simulink model "Q1_2_2"  (R2020b)
settings: Solver=VariableStepAuto  StartTime=0.0  StopTime=20.0  RelTol=1e-3
libraries: simulink x2
settings Model: Creator=kushagrakhatwani  LastModifiedBy=kushagrakhatwani

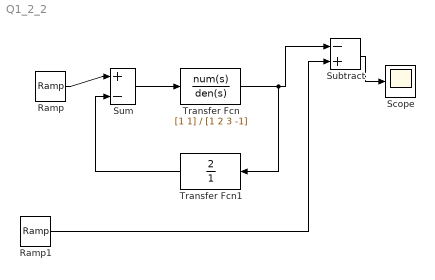
== system Q1_2_2 ==
  Ramp : simulink/Sources/Ramp  slope=1  start=0  InitialOutput=0
  Ramp1 : simulink/Sources/Ramp  slope=1  start=0  InitialOutput=0
  Scope : Scope
  Subtract : Sum  Inputs=-+
  Sum : Sum  Inputs=|+-
  Transfer Fcn : TransferFcn  Numerator=[1 1]  Denominator=[1 2 3 -1]
  Transfer Fcn1 : TransferFcn  Numerator=[2]  Denominator=[1]
  wires:
  Transfer Fcn1/1 -> Sum/2
  Ramp/1 -> Sum/1
  Sum/1 -> Transfer Fcn/1
  Transfer Fcn/1 -> Transfer Fcn1/1, Subtract/1
  Ramp1/1 -> Subtract/2
  Subtract/1 -> Scope/1
